simulink library "lib_Transmission"  (R2017b)
settings: Solver=VariableStepAuto  StartTime=0.0  StopTime=10.0  RelTol=1e-3
undefined symbols (not defined in the file): Engine, gb, Gearbox, Loss, Ratio, Spd
libraries: simulink x5
settings Model: Creator=Vraj M  LastModifiedBy=Lyu19
settings CodeAppCC: StateflowObjectComments=on

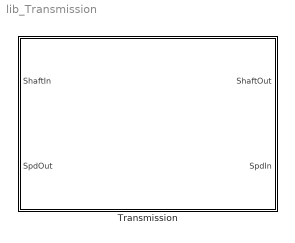
== system lib_Transmission ==
  Transmission : Subsystem
      mask Display:
      | image('Images\Trans.png')
      | color('red');
      | port_label('Input',1,'ShaftIn')
      | port_label('Input',2,'SpdOut')
      | port_label('Output',1,'ShaftOut')
      | port_label('Output',2,'SpdIn')

== system lib_Transmission/Transmission ==
  ShaftIn : Inport
  SpdOut : Inport  Port=2
  Inputs : Subsystem  AncestorBlock=lib_DCDC/DC-DC Converter/Inputs
  Outputs : Subsystem  AncestorBlock=lib_DCDC/DC-DC Converter/Outputs
  Soft TCM : Subsystem
      mask Display: image('softECU.jpg')
  Transmission Plant : Subsystem
      mask Display:
      | image('Images\Trans.png')
      | color('red');
      | port_label('Input',2,'ShaftIn')
      | port_label('Input',3,'SpdOut')
      | port_label('Output',2,'ShaftOut')
      | port_label('Output',3,'SpdIn')
  ShaftOut : Outport
  SpdIn : Outport  Port=2
  wires:
  Transmission Plant/3(TorqConvSpdIn) -> SpdIn/1
  Transmission Plant/2(GearboxShaftOut) -> ShaftOut/1
  SpdOut/1 -> Transmission Plant/3(GearboxSpdOut)
  ShaftIn/1 -> Transmission Plant/2(TorqConvShaftIn)
  Soft TCM/1(Out) -> Outputs/1(Outputs)
  Inputs/1(Inputs) -> Soft TCM/1(In)
  Transmission Plant/1(Out1) -> Soft TCM/2(In1)  "Sensors_to_TCM"
  Soft TCM/2(Out1) -> Transmission Plant/1("In1 ")  "TCM_to_Actuators"

== system lib_Transmission/Transmission/Inputs ==
  Analog_fromHCU : Subsystem
  Bus Creator1 : BusCreator  Inputs=3
  CAN_fromHCU : Subsystem
  Digital_fromHCU : Subsystem
  Inputs : Outport
  wires:
  Digital_fromHCU/1(Outputs) -> Bus Creator1/2  "Digital"
  CAN_fromHCU/1(Outputs) -> Bus Creator1/1  "CAN"
  Bus Creator1/1 -> Inputs/1
  Analog_fromHCU/1(Outputs) -> Bus Creator1/3

== system lib_Transmission/Transmission/Outputs ==
  Outputs : Inport
  tag scope: TCM_to_HCU=global
  wires:
  Outputs/1 -> [TCM_to_HCU]  "TCM_CAN"

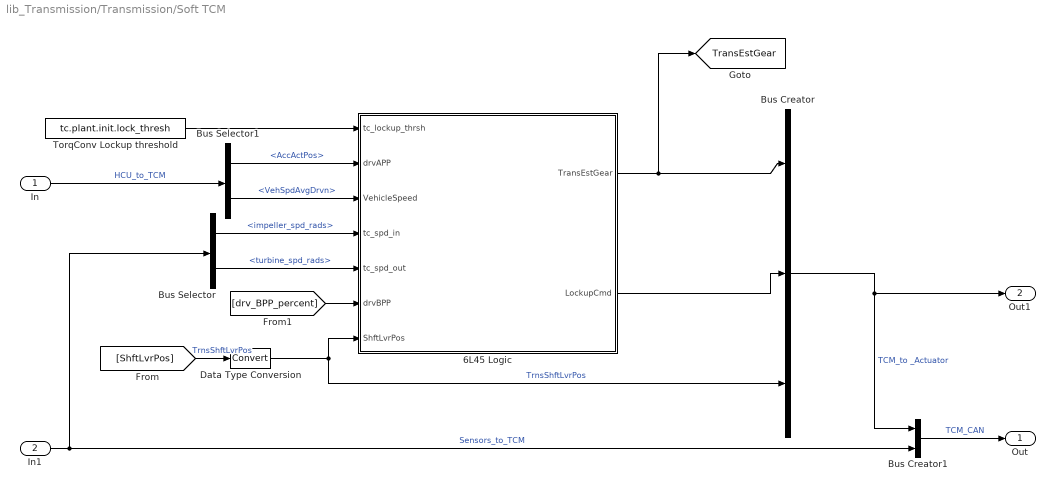
== system lib_Transmission/Transmission/Soft TCM ==
  In : Inport
  In1 : Inport  Port=2
  6L45 Logic : Stateflow chart  TreatAsAtomicUnit=on
  Bus Creator : BusCreator  Inputs=3
  Bus Creator1 : BusCreator  Inputs=2
  Bus Selector : BusSelector  OutputSignals=impeller_spd_rads,turbine_spd_rads
  Bus Selector1 : BusSelector  OutputSignals=CAN.PPEI_Engine_General_Status_1.AccActPos,CAN.PPEI_Vehicle_Speed_and_Distance.VehSpdAvgDrvn
  Data Type Conversion : DataTypeConversion
  TorqConv Lockup threshold : Constant  Value=tc.plant.init.lock_thresh
  Out : Outport
  Out1 : Outport  Port=2
  tag scope: TransEstGear=global
  wires:
  TorqConv Lockup threshold/1 -> 6L45 Logic/1(tc_lockup_thrsh)
  6L45 Logic/1(TransEstGear) -> [TransEstGear], Bus Creator/1
  Data Type Conversion/1 -> Bus Creator/3, 6L45 Logic/7(ShftLvrPos)  "TrnsShftLvrPos"
  In1/1 -> Bus Selector/1, Bus Creator1/2  "Sensors_to_TCM"
  Bus Creator1/1 -> Out/1  "TCM_CAN"
  In/1 -> Bus Selector1/1  "HCU_to_TCM"
  Bus Selector/2 -> 6L45 Logic/5(tc_spd_out)  "<turbine_spd_rads>"
  Bus Selector/1 -> 6L45 Logic/4(tc_spd_in)  "<impeller_spd_rads>"
  Bus Selector1/2 -> 6L45 Logic/3(VehicleSpeed)  "<VehSpdAvgDrvn>"
  Bus Selector1/1 -> 6L45 Logic/2(drvAPP)  "<AccActPos>"
  Bus Creator/1 -> Out1/1, Bus Creator1/1  "TCM_to _Actuator"
  6L45 Logic/2(LockupCmd) -> Bus Creator/2
  [drv_BPP_percent] -> 6L45 Logic/6(drvBPP)
  [ShftLvrPos] -> Data Type Conversion/1  "TrnsShftLvrPos"

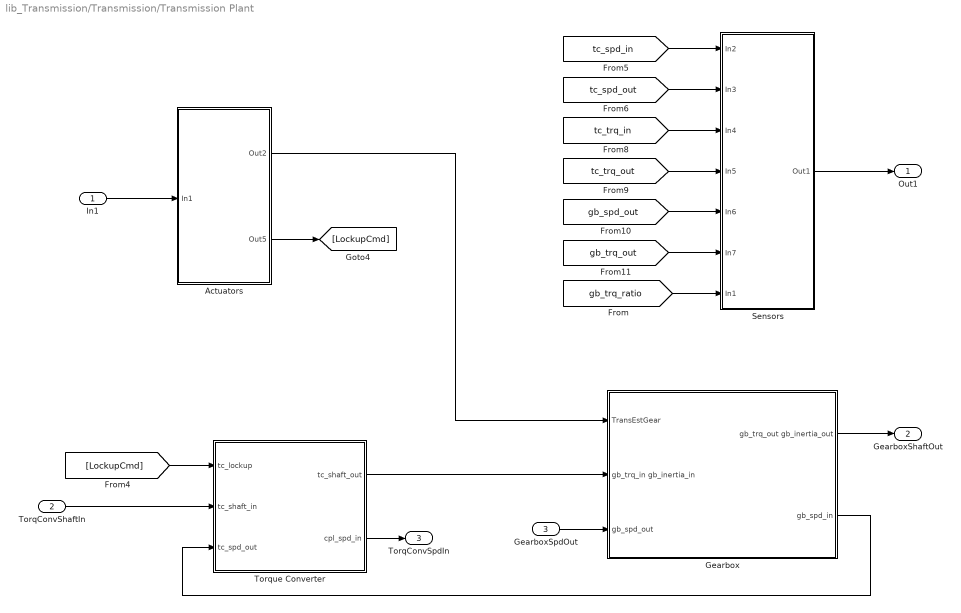
== system lib_Transmission/Transmission/Transmission Plant ==
  "In1 " : Inport
  TorqConvShaftIn : Inport  Port=2
  GearboxSpdOut : Inport  Port=3
  " Actuators" : Subsystem
  Gearbox : Subsystem
      mask Display:
      | image('Images\Gearbox.jpg')
      | color('red');
      | port_label('Input',1,'Gear');
      | port_label('Input',2,'ShftIn');
      | port_label('Input',3,'SpdOut');
      | port_label('Output',1,'ShaftOut');
      | port_label('Output',2,'SpdIn');
  Sensors : Subsystem
  Torque Converter : Subsystem
      mask Display:
      | image('Images\TorqConv.jpg')
      | color('red');
      | port_label('Input',2,'ShaftIn');
      | port_label('Input',3,'SpdOut');
      | port_label('Output',1,'ShaftOut');
      | port_label('Output',2,'SpdIn');
  Out1 : Outport
  GearboxShaftOut : Outport  Port=2
  TorqConvSpdIn : Outport  Port=3
  wires:
  [tc_trq_out] -> Sensors/4(In5)
  [gb_spd_out] -> Sensors/5(In6)
  [gb_trq_out] -> Sensors/6(In7)
  [tc_spd_out] -> Sensors/2(In3)
  [tc_spd_in] -> Sensors/1(In2)
  [tc_trq_in] -> Sensors/3(In4)
  " Actuators"/2(Out5) -> [LockupCmd]
  "In1 "/1 -> " Actuators"/1(In1)
  Sensors/1(Out1) -> Out1/1
  [gb_trq_ratio] -> Sensors/7(In1)
  Torque Converter/2(cpl_spd_in) -> TorqConvSpdIn/1
  Gearbox/2(gb_spd_in) -> Torque Converter/3(tc_spd_out)
  TorqConvShaftIn/1 -> Torque Converter/2(tc_shaft_in)
  Gearbox/1(gb_trq_out gb_inertia_out) -> GearboxShaftOut/1
  " Actuators"/1(Out2) -> Gearbox/1(TransEstGear)
  Torque Converter/1(tc_shaft_out) -> Gearbox/2(gb_trq_in gb_inertia_in)
  GearboxSpdOut/1 -> Gearbox/3(gb_spd_out)
  [LockupCmd] -> Torque Converter/1(tc_lockup)

== system lib_Transmission/Transmission/Inputs/Analog_fromHCU ==
  Outputs : Outport
  wires:
  [Analog] -> Outputs/1

== system lib_Transmission/Transmission/Inputs/CAN_fromHCU ==
  Outputs : Outport
  wires:
  [HCU_to_VEH_CAN] -> Outputs/1

== system lib_Transmission/Transmission/Inputs/Digital_fromHCU ==
  Outputs : Outport
  wires:
  [Digital] -> Outputs/1

== system lib_Transmission/Transmission/Soft TCM/6L45 Logic/Gearbox_Control.Shift_Schedule.PlotShiftSchedule ==
  f : TriggerPort  TriggerType=function-call  VariantControl=Variant
      settings: CopyFcn=Stateflow.SLINSF.SimulinkMan.removeBlockPreDeleteFcn  PreDeleteFcn=Stateflow.SLINSF.SimulinkMan.unsafePredeleteFcn
  Subsystem : Subsystem
      settings: OpenFcn=|
      | figure;
      | PlotGearShiftSchedule(Gearbox.L45.PedalPositions,Gearbox.L45.UpShiftSpeeds,Gearbox.L45.DownShiftSpeeds,'6L45')
      mask Display: disp('Plot')

== system lib_Transmission/Transmission/Soft TCM/6L45 Logic/Gearbox_Control.Shift_Schedule.calc_down ==
  Gear : Inport
  APP : Inport  Port=2
  f : TriggerPort  TriggerType=function-call  VariantControl=Variant
      settings: CopyFcn=Stateflow.SLINSF.SimulinkMan.removeBlockPreDeleteFcn  PreDeleteFcn=Stateflow.SLINSF.SimulinkMan.unsafePredeleteFcn
  Calculate Downshift Threshold : Lookup2D  RowIndex=gb.ctrl.dmd.init.gear_dnshift.idx1_lin_accel  ColumnIndex=[2,3,4,5,6,7,8]  Table=gb.ctrl.dmd.init.gear_dnshift.map'  LookUpMeth=Interpolation-Use End Values
  down_th : Outport
  wires:
  APP/1 -> Calculate Downshift Threshold/1
  Gear/1 -> Calculate Downshift Threshold/2
  Calculate Downshift Threshold/1 -> down_th/1

== system lib_Transmission/Transmission/Soft TCM/6L45 Logic/Gearbox_Control.Shift_Schedule.calc_up ==
  Gear : Inport
  APP : Inport  Port=2
  f : TriggerPort  TriggerType=function-call  VariantControl=Variant
      settings: CopyFcn=Stateflow.SLINSF.SimulinkMan.removeBlockPreDeleteFcn  PreDeleteFcn=Stateflow.SLINSF.SimulinkMan.unsafePredeleteFcn
  Calculate Upshift Threshold : Lookup2D  RowIndex=gb.ctrl.dmd.init.gear_upshift.idx1_lin_accel  ColumnIndex=[1,2,3,4,5,6,7]  Table=gb.ctrl.dmd.init.gear_upshift.map'  LookUpMeth=Interpolation-Use End Values
  up_th : Outport
  wires:
  Gear/1 -> Calculate Upshift Threshold/2
  APP/1 -> Calculate Upshift Threshold/1
  Calculate Upshift Threshold/1 -> up_th/1

== system lib_Transmission/Transmission/Soft TCM/6L45 Logic/Torque_Converter_Control.calc_lockup ==
  Gear : Inport
  APP : Inport  Port=2
  f : TriggerPort  TriggerType=function-call  VariantControl=Variant
      settings: CopyFcn=Stateflow.SLINSF.SimulinkMan.removeBlockPreDeleteFcn  PreDeleteFcn=Stateflow.SLINSF.SimulinkMan.unsafePredeleteFcn
  Calculate Lockup Threshold : Lookup2D  RowIndex=cpl.ctrl.init.trqconv_lockup.idx1_lin_accel  ColumnIndex=cpl.ctrl.init.trqconv_lockup.idx2_gear  Table=cpl.ctrl.init.trqconv_lockup.map  LookUpMeth=Interpolation-Use End Values
  lockup_th : Outport
  wires:
  Gear/1 -> Calculate Lockup Threshold/2
  APP/1 -> Calculate Lockup Threshold/1
  Calculate Lockup Threshold/1 -> lockup_th/1

== system lib_Transmission/Transmission/Soft TCM/6L45 Logic/Torque_Converter_Control.calc_unlock ==
  Gear : Inport
  APP : Inport  Port=2
  f : TriggerPort  TriggerType=function-call  VariantControl=Variant
      settings: CopyFcn=Stateflow.SLINSF.SimulinkMan.removeBlockPreDeleteFcn  PreDeleteFcn=Stateflow.SLINSF.SimulinkMan.unsafePredeleteFcn
  Calculate Unlock Threshold : Lookup2D  RowIndex=cpl.ctrl.init.trqconv_unlock.idx1_lin_accel  ColumnIndex=cpl.ctrl.init.trqconv_unlock.idx2_gear  Table=cpl.ctrl.init.trqconv_unlock.map  LookUpMeth=Interpolation-Use End Values
  unlock_th : Outport
  wires:
  Gear/1 -> Calculate Unlock Threshold/2
  APP/1 -> Calculate Unlock Threshold/1
  Calculate Unlock Threshold/1 -> unlock_th/1

== system lib_Transmission/Transmission/Transmission Plant/ Actuators ==
  In1 : Inport
  Bus Selector : BusSelector  OutputSignals=TransEstGear,LockupCmd
  Out2 : Outport
  Out5 : Outport  Port=2
  wires:
  Bus Selector/2 -> Out5/1  "<LockupCmd>"
  Bus Selector/1 -> Out2/1  "<TransEstGear>"
  In1/1 -> Bus Selector/1

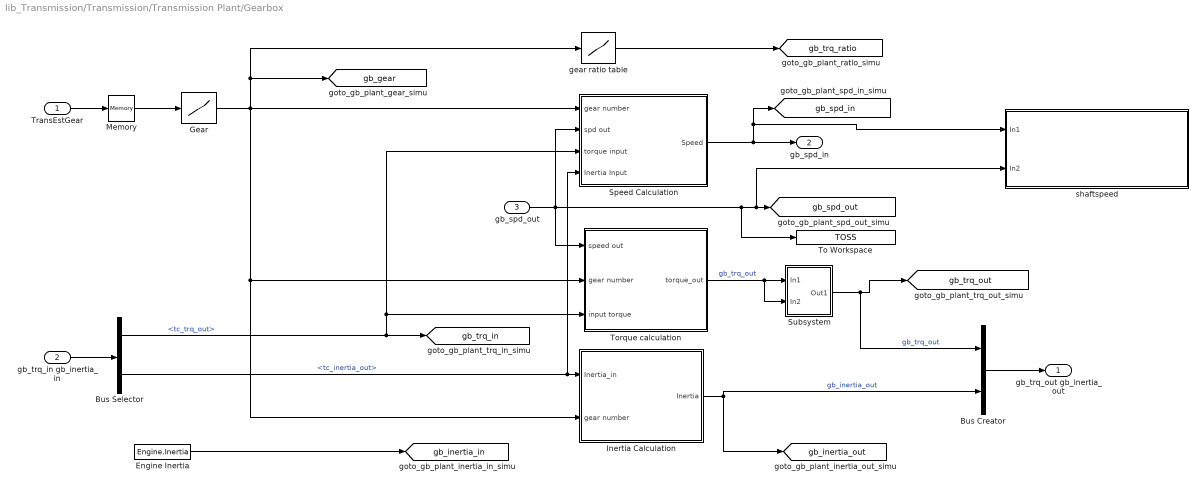
== system lib_Transmission/Transmission/Transmission Plant/Gearbox ==
  TransEstGear : Inport
  gb_trq_in gb_inertia_in : Inport  Port=2
  gb_spd_out : Inport  Port=3
  Bus Creator : BusCreator  Inputs=2
  Bus Selector : BusSelector  OutputSignals=tc_trq_out,tc_inertia_out
  Engine Inertia : Constant  Value=Engine.Inertia
  Gear : Lookup  InputValues=gb.plant.init.gear.idx1_shifter  Table=gb.plant.init.gear.idx2_gear  LookUpMeth=Interpolation-Use End Values  OutDataTypeStr=double  SaturateOnIntegerOverflow=on
  Inertia Calculation : Subsystem
  Memory : Memory
  Speed Calculation : Subsystem
  Subsystem : Subsystem
  To Workspace : ToWorkspace  VariableName=TOSS  SampleTime=-1
  Torque calculation : Subsystem
  gear ratio table : Lookup  InputValues=gb.plant.init.ratio.idx1_gear  Table=gb.plant.init.ratio.map  LookUpMeth=Interpolation-Use End Values  SaturateOnIntegerOverflow=on
  "shaftspeed " : Subsystem
  gb_trq_out gb_inertia_out : Outport
  gb_spd_in : Outport  Port=2
  tag scope: gb_gear=global, gb_inertia_in=global, gb_inertia_out=global, gb_spd_in=global, gb_spd_out=global, gb_trq_in=global, gb_trq_out=global, gb_trq_ratio=global
  wires:
  TransEstGear/1 -> Memory/1
  Bus Selector/1 -> [gb_trq_in], Speed Calculation/3(torque input), Torque calculation/3(" input torque")  "<tc_trq_out>"
  Gear/1 -> Speed Calculation/1(gear number), [gb_gear], gear ratio table/1, Inertia Calculation/2(gear number), Torque calculation/2(gear number)
  gb_spd_out/1 -> Torque calculation/1(speed out), To Workspace/1, "shaftspeed "/2(In2), [gb_spd_out], Speed Calculation/2(spd out)
  gb_trq_in gb_inertia_in/1 -> Bus Selector/1
  Speed Calculation/1(Speed) -> "shaftspeed "/1(In1), [gb_spd_in], gb_spd_in/1
  Inertia Calculation/1(Inertia) -> [gb_inertia_out], Bus Creator/2  "gb_inertia_out"
  Bus Creator/1 -> gb_trq_out gb_inertia_out/1
  gear ratio table/1 -> [gb_trq_ratio]
  Memory/1 -> Gear/1
  Torque calculation/1(torque_out) -> Subsystem/2(In2), Subsystem/1(In1)  "gb_trq_out"
  Subsystem/1(Out1) -> Bus Creator/1, [gb_trq_out]  "gb_trq_out"
  Engine Inertia/1 -> [gb_inertia_in]
  Bus Selector/2 -> Speed Calculation/4(Inertia Input), Inertia Calculation/1(Inertia_in)  "<tc_inertia_out>"

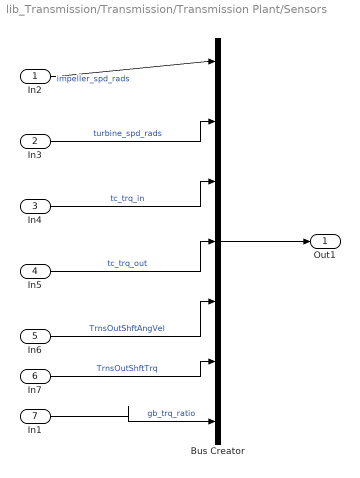
== system lib_Transmission/Transmission/Transmission Plant/Sensors ==
  In2 : Inport
  In3 : Inport  Port=2
  In4 : Inport  Port=3
  In5 : Inport  Port=4
  In6 : Inport  Port=5
  In7 : Inport  Port=6
  In1 : Inport  Port=7
  Bus Creator : BusCreator  Inputs=7
  Out1 : Outport
  wires:
  In7/1 -> Bus Creator/6  "TrnsOutShftTrq"
  In6/1 -> Bus Creator/5  "TrnsOutShftAngVel"
  In3/1 -> Bus Creator/2  "turbine_spd_rads"
  In5/1 -> Bus Creator/4  "tc_trq_out"
  In4/1 -> Bus Creator/3  "tc_trq_in"
  In2/1 -> Bus Creator/1  "impeller_spd_rads"
  Bus Creator/1 -> Out1/1
  In1/1 -> Bus Creator/7  "gb_trq_ratio"

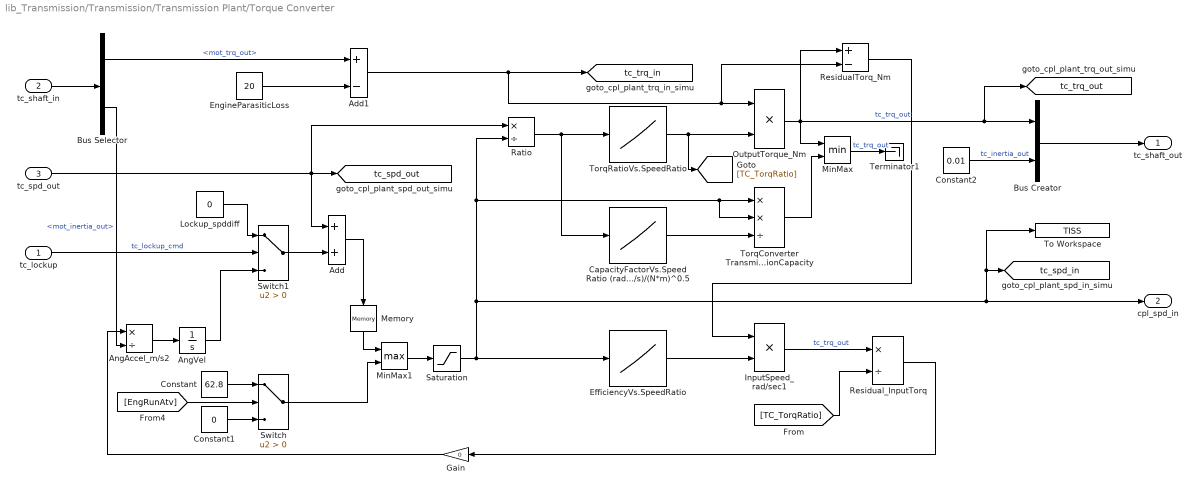
== system lib_Transmission/Transmission/Transmission Plant/Torque Converter ==
  tc_lockup : Inport
  tc_shaft_in : Inport  Port=2
  tc_spd_out : Inport  Port=3
  Add : Sum
  Add1 : Sum  Inputs=+-
  AngAccel_m/s2 : Product  Inputs=*/
  AngVel : Integrator
  Bus Creator : BusCreator  Inputs=2
  Bus Selector : BusSelector  OutputSignals=mot_trq_out,mot_inertia_out
  CapacityFactorVs.SpeedRatio (rad/s)/(N*m)^0.5 : Lookup_n-D  NumberOfTableDimensions=1  BreakpointsForDimension1=[0 0.50 0.60 0.70 0.80 0.87 0.92 0.94 0.96 0.97]  Table=[12.2938 12.8588 13.1452 13.6285 14.6163 16.2675 19.3503 22.1046 29.9986 50.00]  InternalRulePriority=Speed  RndMeth=Simplest  InputSameDT=on
  Constant : Constant  Value=62.8
  Constant1 : Constant  Value=0
  Constant2 : Constant  Value=0.01
  EfficiencyVs.SpeedRatio : Lookup_n-D  NumberOfTableDimensions=1  BreakpointsForDimension1=[0 0.25 0.50 0.60 0.70 0.80 0.87 0.92 0.94 0.96 0.97 1.0]  Table="[0.10 0.50 0.70 0.8 0.8 0.80  0.85 0.87 0.91 0.95 0.96 0.96]"  InternalRulePriority=Speed  RndMeth=Simplest  InputSameDT=on
  EngineParasiticLoss : Constant  Value=20
  Gain : Gain  Gain=0
  InputSpeed_rad/sec1 : Product  Inputs=**
  Lockup_spddiff : Constant  Value=0
  Memory : Memory  InitialCondition=1
  MinMax : MinMax  Inputs=2
  MinMax1 : MinMax  Function=max  Inputs=2
  OutputTorque_Nm : Product  Inputs=**
  Ratio : Product  Inputs=*/
  ResidualTorq_Nm : Sum  Inputs=+-
  Residual_InputTorq : Product  Inputs=*/
  Saturation : Saturate  UpperLimit=1100  LowerLimit=1
  Switch : Switch  Criteria=u2 > Threshold
  Switch1 : Switch  Criteria=u2 > Threshold
  Terminator1 : Terminator
  To Workspace : ToWorkspace  VariableName=TISS  SampleTime=-1
  TorqConverter TransmissionCapacity : Product  Inputs=**/
  TorqRatioVs.SpeedRatio : Lookup_n-D  NumberOfTableDimensions=1  BreakpointsForDimension1=[0 0.50 0.60 0.70 0.80 0.87 0.92 0.94 0.96 0.97]  Table=[2.2320 1.5462 1.4058 1.2746 1.1528 1.0732 1.0192 0.9983 0.9983 0.9983]  InternalRulePriority=Speed  RndMeth=Simplest  InputSameDT=on
  tc_shaft_out : Outport
  cpl_spd_in : Outport  Port=2
  tag scope: tc_spd_in=global, tc_spd_out=global, tc_trq_in=global, tc_trq_out=global
  wires:
  Add1/1 -> [tc_trq_in], ResidualTorq_Nm/2, OutputTorque_Nm/1
  Constant2/1 -> Bus Creator/2  "tc_inertia_out"
  tc_shaft_in/1 -> Bus Selector/1
  Bus Creator/1 -> tc_shaft_out/1
  Bus Selector/2 -> AngAccel_m/s2/2  "<mot_inertia_out>"
  tc_lockup/1 -> Switch1/2  "tc_lockup_cmd"
  TorqRatioVs.SpeedRatio/1 -> OutputTorque_Nm/2, [TC_TorqRatio]
  CapacityFactorVs.SpeedRatio (rad/s)/(N*m)^0.5/1 -> TorqConverter TransmissionCapacity/3
  Ratio/1 -> CapacityFactorVs.SpeedRatio (rad/s)/(N*m)^0.5/1, TorqRatioVs.SpeedRatio/1
  Saturation/1 -> Ratio/2, TorqConverter TransmissionCapacity/2, TorqConverter TransmissionCapacity/1, [tc_spd_in], To Workspace/1, cpl_spd_in/1, EfficiencyVs.SpeedRatio/1
  EfficiencyVs.SpeedRatio/1 -> InputSpeed_rad/sec1/2
  TorqConverter TransmissionCapacity/1 -> MinMax/2
  [TC_TorqRatio] -> Residual_InputTorq/2
  ResidualTorq_Nm/1 -> InputSpeed_rad/sec1/1
  InputSpeed_rad/sec1/1 -> Residual_InputTorq/1  "tc_trq_out"
  AngAccel_m/s2/1 -> AngVel/1
  AngVel/1 -> Switch1/3
  Memory/1 -> MinMax1/1
  EngineParasiticLoss/1 -> Add1/2
  Residual_InputTorq/1 -> Gain/1
  OutputTorque_Nm/1 -> ResidualTorq_Nm/1, Bus Creator/1, [tc_trq_out], MinMax/1  "tc_trq_out"
  MinMax/1 -> Terminator1/1  "tc_trq_out"
  tc_spd_out/1 -> Ratio/1, [tc_spd_out], Add/1
  Add/1 -> Memory/1
  Gain/1 -> AngAccel_m/s2/1
  MinMax1/1 -> Saturation/1
  Switch/1 -> MinMax1/2
  [EngRunAtv] -> Switch/2
  Constant/1 -> Switch/1
  Constant1/1 -> Switch/3
  Bus Selector/1 -> Add1/1  "<mot_trq_out>"
  Switch1/1 -> Add/2
  Lockup_spddiff/1 -> Switch1/1

== system lib_Transmission/Transmission/Soft TCM/6L45 Logic/Gearbox_Control.Shift_Schedule.PlotShiftSchedule/Subsystem ==

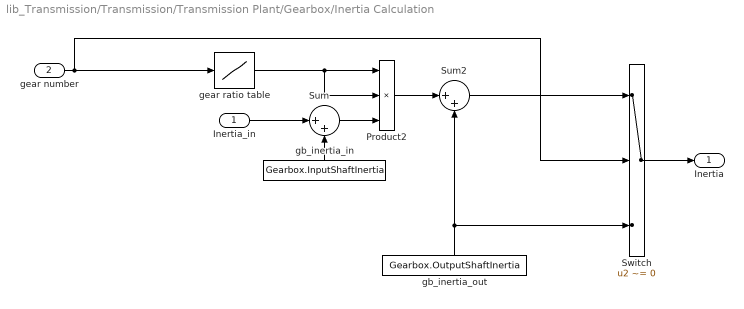
== system lib_Transmission/Transmission/Transmission Plant/Gearbox/Inertia Calculation ==
  Inertia_in : Inport
  gear number : Inport  Port=2
  Product2 : Product  Inputs=3  SaturateOnIntegerOverflow=on  InputSameDT=on  OutDataTypeStr=Inherit: Same as first input
  Sum : Sum  Inputs=|++  SaturateOnIntegerOverflow=on  InputSameDT=on  OutDataTypeStr=Inherit: Same as first input
  Sum2 : Sum  Inputs=|++  SaturateOnIntegerOverflow=on  InputSameDT=on  OutDataTypeStr=Inherit: Same as first input
  Switch : Switch  Criteria=u2 ~= 0  Threshold=0.5  SaturateOnIntegerOverflow=on  InputSameDT=on
  gb_inertia_in : Constant  Value=Gearbox.InputShaftInertia
  gb_inertia_out : Constant  Value=Gearbox.OutputShaftInertia
  gear ratio table : Lookup  InputValues=gb.plant.init.ratio.idx1_gear  Table=gb.plant.init.ratio.map  OutDataTypeStr=double  SaturateOnIntegerOverflow=on
  Inertia : Outport
  wires:
  gear ratio table/1 -> Product2/1, Product2/2
  Sum2/1 -> Switch/1
  Inertia_in/1 -> Sum/1
  Product2/1 -> Sum2/1
  gb_inertia_in/1 -> Sum/2
  Sum/1 -> Product2/3
  gb_inertia_out/1 -> Sum2/2, Switch/3
  gear number/1 -> Switch/2, gear ratio table/1
  Switch/1 -> Inertia/1

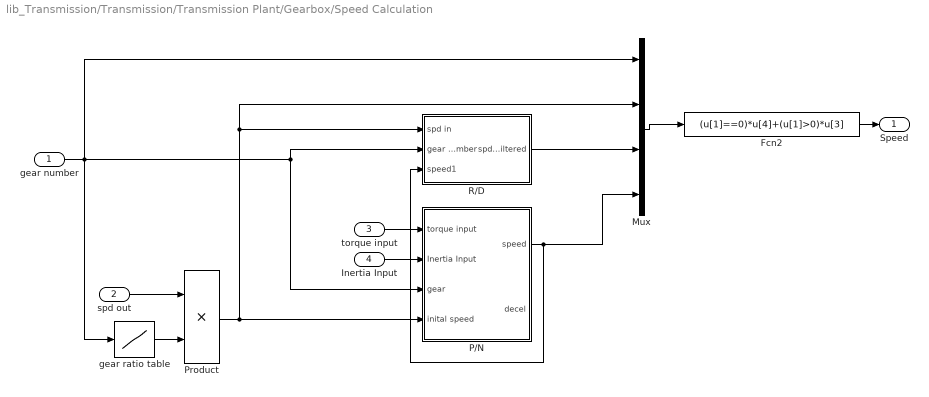
== system lib_Transmission/Transmission/Transmission Plant/Gearbox/Speed Calculation ==
  gear number : Inport
  spd out : Inport  Port=2
  torque input : Inport  Port=3
  Inertia Input : Inport  Port=4
  Fcn2 : Fcn  Expr=(u[1]==0)*u[4]+(u[1]>0)*u[3]
  Mux : Mux
  P/N : Subsystem
  Product : Product  SaturateOnIntegerOverflow=on  InputSameDT=on  OutDataTypeStr=Inherit: Same as first input
  R/D : Subsystem
  gear ratio table : Lookup  InputValues=gb.plant.init.ratio.idx1_gear  Table=gb.plant.init.ratio.map  SaturateOnIntegerOverflow=on
  Speed : Outport
  wires:
  Mux/1 -> Fcn2/1
  gear number/1 -> Mux/1, P/N/3(gear), R/D/2(gear number), gear ratio table/1
  torque input/1 -> P/N/1(torque input)
  Inertia Input/1 -> P/N/2(Inertia Input)
  spd out/1 -> Product/1
  gear ratio table/1 -> Product/2
  Product/1 -> Mux/2, R/D/1(spd in), P/N/4(inital speed)
  P/N/1(speed) -> Mux/4, R/D/3(speed1)
  R/D/1(spd in filtered) -> Mux/3
  Fcn2/1 -> Speed/1

== system lib_Transmission/Transmission/Transmission Plant/Gearbox/Subsystem ==
  In1 : Inport
  In2 : Inport  Port=2
  Add : Sum
  Constant : Constant  Value=200
  Switch2 : Switch  Criteria=u2 > Threshold
  Out1 : Outport
  wires:
  Add/1 -> Switch2/1
  Constant/1 -> Add/1
  [Brk_Flt] -> Switch2/2
  In2/1 -> Switch2/3
  In1/1 -> Add/2
  Switch2/1 -> Out1/1

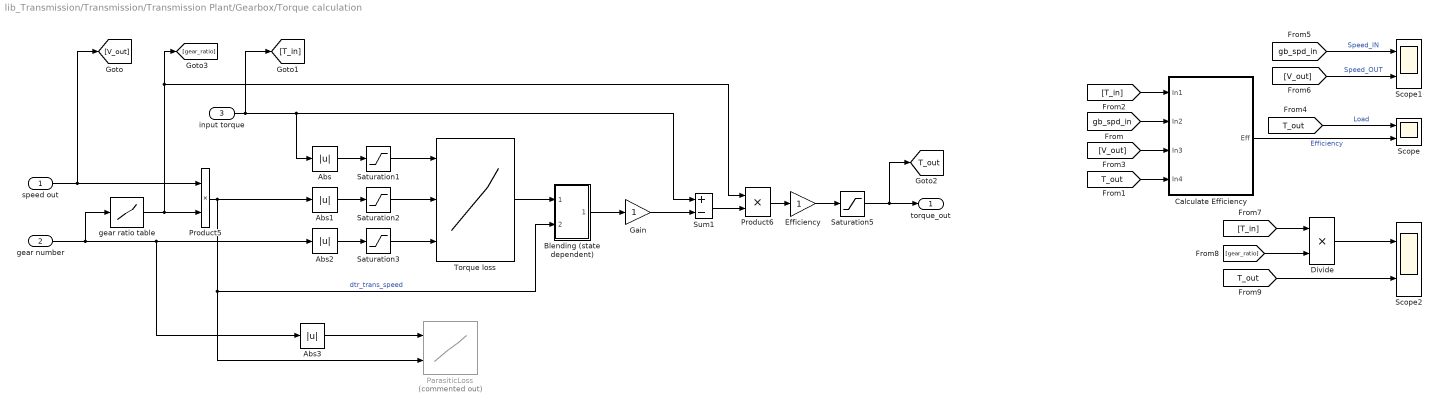
== system lib_Transmission/Transmission/Transmission Plant/Gearbox/Torque calculation ==
  speed out : Inport
  gear number : Inport  Port=2
  " input torque" : Inport  Port=3
  Abs : Abs  SaturateOnIntegerOverflow=on
  Abs1 : Abs  SaturateOnIntegerOverflow=on
  Abs2 : Abs  SaturateOnIntegerOverflow=on
  Abs3 : Abs
  Blending (state dependent) : Subsystem  mask(State dependent blending){xl=-gb.plant.init.spd_thr, yl=-1, xc=0, yc=0, xr=gb.plant.init.spd_thr, yr=1}
      mask prompts: xl "Left point (x):"; yl "Left point (y):"; xc "Center point (x):"; yc "Center point (y):"; xr "Right point (x):"; yr "Right point (y):"
      mask help: This block implements state dependent smoothing/blending. IMPORTANT: See help menu.
      mask Help: The output equals the product of the first input and a "hat" function defined by the three points specified in the dialog box.  The second input forms the argument to the hat function.\n\nIMPORTANT: A divide by zero error will result if first coordinates of the three points specified for the hat function are NOT distinct.
      mask Display: plot([-1 1 3 6 8], [1.5 1.5 0.5 4.0 4.0])
  Calculate Efficiency : Subsystem
  Divide : Product  Inputs=**
  Efficiency : Gain
  Gain : Gain
  ParasiticLoss : Lookup_n-D  Commented=on  BreakpointsForDimension1=Ratio  BreakpointsForDimension2=Spd  Table=Loss  InternalRulePriority=Speed  RndMeth=Simplest  InputSameDT=on
  Product5 : Product  SaturateOnIntegerOverflow=on  InputSameDT=on  OutDataTypeStr=Inherit: Same as first input
  Product6 : Product  SaturateOnIntegerOverflow=on  InputSameDT=on  OutDataTypeStr=Inherit: Same as first input
  Saturation1 : Saturate  UpperLimit=inf  LowerLimit=min( gb.plant.init.trq_loss.idx1_trq )
  Saturation2 : Saturate  UpperLimit=inf  LowerLimit=min( gb.plant.init.trq_loss.idx2_spd )
  Saturation3 : Saturate  UpperLimit=8  LowerLimit=1
  Saturation5 : Saturate  UpperLimit=inf  LowerLimit=min( gb.plant.init.trq_loss.idx1_trq )
  Scope : Scope  NumInputPorts=2
  Scope1 : Scope  NumInputPorts=2
  Scope2 : Scope  NumInputPorts=2
  Sum1 : Sum  Inputs=+-  SaturateOnIntegerOverflow=on  InputSameDT=on  OutDataTypeStr=Inherit: Same as first input
  Torque loss : Lookup_n-D  NumberOfTableDimensions=3  BreakpointsForDimension1=gb.plant.init.trq_loss.idx1_trq  BreakpointsForDimension2=gb.plant.init.trq_loss.idx2_spd  BreakpointsForDimension3=gb.plant.init.trq_loss.idx3_gear  Table=gb.plant.init.trq_loss.map
  gear ratio table : Lookup  InputValues=gb.plant.init.ratio.idx1_gear  Table=gb.plant.init.ratio.map  SaturateOnIntegerOverflow=on
  torque_out : Outport
  tag scope: T_out=global
  wires:
  Saturation2/1 -> Torque loss/2
  Saturation1/1 -> Torque loss/1
  Abs/1 -> Saturation1/1
  Product5/1 -> ParasiticLoss/2, Blending (state dependent)/2(Control (state)), Abs1/1  "dtr_trans_speed"
  Abs1/1 -> Saturation2/1
  speed out/1 -> [V_out], Product5/1
  Product6/1 -> Efficiency/1
  Blending (state dependent)/1(Output) -> Gain/1
  Sum1/1 -> Product6/2
  " input torque"/1 -> [T_in], Sum1/1, Abs/1
  gear number/1 -> Abs3/1, Abs2/1, gear ratio table/1
  gear ratio table/1 -> Product5/2, [gear_ratio], Product6/1
  Abs2/1 -> Saturation3/1
  Saturation3/1 -> Torque loss/3
  Abs3/1 -> ParasiticLoss/1
  Efficiency/1 -> Saturation5/1
  Gain/1 -> Sum1/2
  Torque loss/1 -> Blending (state dependent)/1(Input)
  [T_in] -> Calculate Efficiency/1(In1)
  [gb_spd_in] -> Calculate Efficiency/2(In2)
  [T_out] -> Calculate Efficiency/4(In4)
  Calculate Efficiency/1(Eff) -> Scope/2  "Efficiency"
  [V_out] -> Calculate Efficiency/3(In3)
  [T_out] -> Scope/1  "Load"
  [gb_spd_in] -> Scope1/1  "Speed_IN"
  [V_out] -> Scope1/2  "Speed_OUT"
  [T_in] -> Divide/1
  [gear_ratio] -> Divide/2
  Divide/1 -> Scope2/1
  [T_out] -> Scope2/2
  Saturation5/1 -> torque_out/1, [T_out]

== system lib_Transmission/Transmission/Transmission Plant/Gearbox/shaftspeed  ==
  In1 : Inport
  In2 : Inport  Port=2
  Gain : Gain  Gain=30/pi
  Gain1 : Gain  Gain=30/pi
  Rate Transition1 : RateTransition  OutPortSampleTime=1
  Rate Transition7 : RateTransition  OutPortSampleTime=1
  To Workspace3 : ToWorkspace  VariableName=TrnsOutShftAngVel  SampleTime=-1
  To Workspace4 : ToWorkspace  VariableName=TrnTrbAngVl  SampleTime=-1
  wires:
  In2/1 -> Gain1/1
  In1/1 -> Gain/1
  Gain/1 -> Rate Transition7/1
  Rate Transition7/1 -> To Workspace4/1
  Rate Transition1/1 -> To Workspace3/1
  Gain1/1 -> Rate Transition1/1

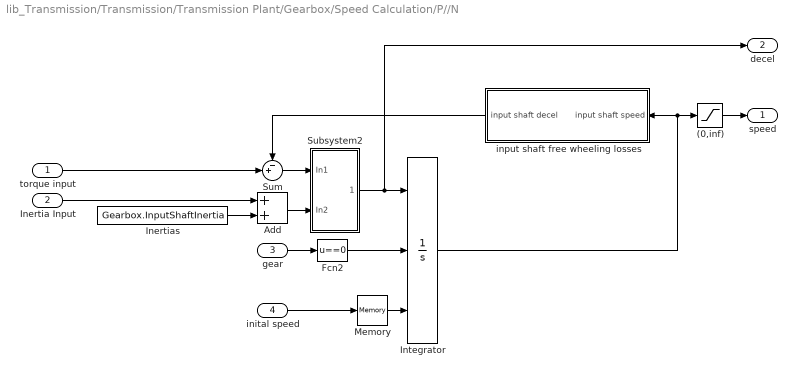
== system lib_Transmission/Transmission/Transmission Plant/Gearbox/Speed Calculation/P//N ==
  torque input : Inport
  Inertia Input : Inport  Port=2
  gear : Inport  Port=3
  inital speed : Inport  Port=4
  (0,inf) : Saturate  UpperLimit=1100  LowerLimit=0
  Add : Sum
  Fcn2 : Fcn  Expr=u==0
  Inertias : Constant  Value=Gearbox.InputShaftInertia
  Integrator : Integrator  ExternalReset=rising  InitialConditionSource=external
  Memory : Memory
  Subsystem2 : Subsystem
      mask Display: disp('divider')
  Sum : Sum  Inputs=-+|  SaturateOnIntegerOverflow=on  InputSameDT=on  OutDataTypeStr=Inherit: Same as first input
  input shaft free wheeling losses : Subsystem
  speed : Outport
  decel : Outport  Port=2
  wires:
  Inertia Input/1 -> Add/1
  Subsystem2/1(Out1) -> decel/1, Integrator/1
  Memory/1 -> Integrator/3
  (0,inf)/1 -> speed/1
  torque input/1 -> Sum/2
  Sum/1 -> Subsystem2/1(In1)
  input shaft free wheeling losses/1(input shaft decel) -> Sum/1
  Integrator/1 -> input shaft free wheeling losses/1(input shaft speed), (0,inf)/1
  gear/1 -> Fcn2/1
  inital speed/1 -> Memory/1
  Fcn2/1 -> Integrator/2
  Add/1 -> Subsystem2/2(In2)
  Inertias/1 -> Add/2

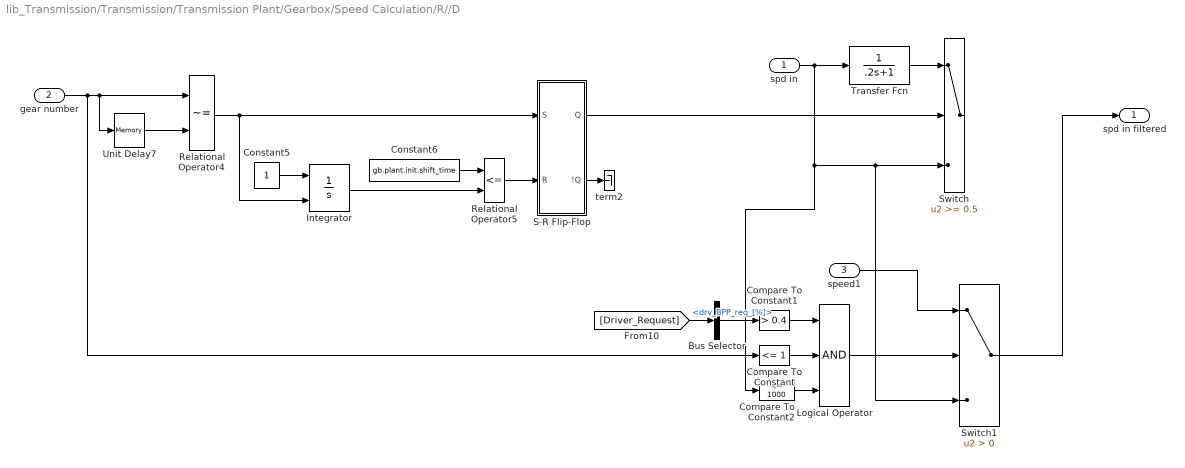
== system lib_Transmission/Transmission/Transmission Plant/Gearbox/Speed Calculation/R//D ==
  spd in : Inport
  gear number : Inport  Port=2
  speed1 : Inport  Port=3
  Bus Selector : BusSelector  OutputSignals=drv_BPP_req_[%]
  Compare To Constant : simulink/Logic and Bit Operations/Compare To Constant  relop=<=  const=1  OutDataTypeStr=boolean
  Compare To Constant1 : simulink/Logic and Bit Operations/Compare To Constant  relop=>  const=0.4  OutDataTypeStr=boolean
  Compare To Constant2 : simulink/Logic and Bit Operations/Compare To Constant  relop=<=  const=1000  OutDataTypeStr=boolean
  Constant5 : Constant
  Constant6 : Constant  Value=gb.plant.init.shift_time
  Integrator : Integrator  ExternalReset=rising
  Logical Operator : Logic  Inputs=3  AllPortsSameDT=off  OutDataTypeStr=boolean
  Relational Operator4 : RelationalOperator  Operator=~=  RndMeth=Nearest  InputSameDT=on
  Relational Operator5 : RelationalOperator  Operator=<=  RndMeth=Nearest  InputSameDT=on
  S-R Flip-Flop : Subsystem  mask(SRFlipFlop){initial_condition=0}
      mask prompts: initial_condition "Initial condition:"
      mask help: S-R Flip Flop Block
  Switch : Switch  Threshold=0.5  SaturateOnIntegerOverflow=on  InputSameDT=on
  Switch1 : Switch  Criteria=u2 > Threshold
  Transfer Fcn : TransferFcn  Denominator=[.2 1]
  Unit Delay7 : Memory
  term2 : Terminator
  spd in filtered : Outport
  wires:
  spd in/1 -> Transfer Fcn/1, Switch/3, Switch1/3, Compare To Constant2/1
  Relational Operator5/1 -> S-R Flip-Flop/2(R)
  S-R Flip-Flop/1(Q) -> Switch/2
  Integrator/1 -> Relational Operator5/2
  Relational Operator4/1 -> S-R Flip-Flop/1(S), Integrator/2
  Unit Delay7/1 -> Relational Operator4/2
  S-R Flip-Flop/2(!Q) -> term2/1
  Constant6/1 -> Relational Operator5/1
  Constant5/1 -> Integrator/1
  gear number/1 -> Compare To Constant/1, Unit Delay7/1, Relational Operator4/1
  [Driver_Request] -> Bus Selector/1
  Bus Selector/1 -> Compare To Constant1/1  "<drv_BPP_req_[%]>"
  Compare To Constant1/1 -> Logical Operator/1
  Compare To Constant/1 -> Logical Operator/2
  Logical Operator/1 -> Switch1/2
  Compare To Constant2/1 -> Logical Operator/3
  Switch1/1 -> spd in filtered/1
  speed1/1 -> Switch1/1
  Transfer Fcn/1 -> Switch/1

== system lib_Transmission/Transmission/Transmission Plant/Gearbox/Torque calculation/Blending (state dependent) ==
  Input : Inport
  Control (state) : Inport  Port=2
  Linear spline : Fcn  Expr=(u<xl)*yl + (xl<=u)*(u<xc)*((yc-yl)*(u-xl)/(xc-xl)+yl) + (xc<=u)*(u<xr)*((yc-yr)*(u-xr)/(xc-xr)+yr) + (xr<=u)*yr
  Product2 : Product  SaturateOnIntegerOverflow=on  InputSameDT=on  OutDataTypeStr=Inherit: Same as first input
  Output : Outport
  wires:
  Control (state)/1 -> Linear spline/1
  Product2/1 -> Output/1
  Linear spline/1 -> Product2/2
  Input/1 -> Product2/1

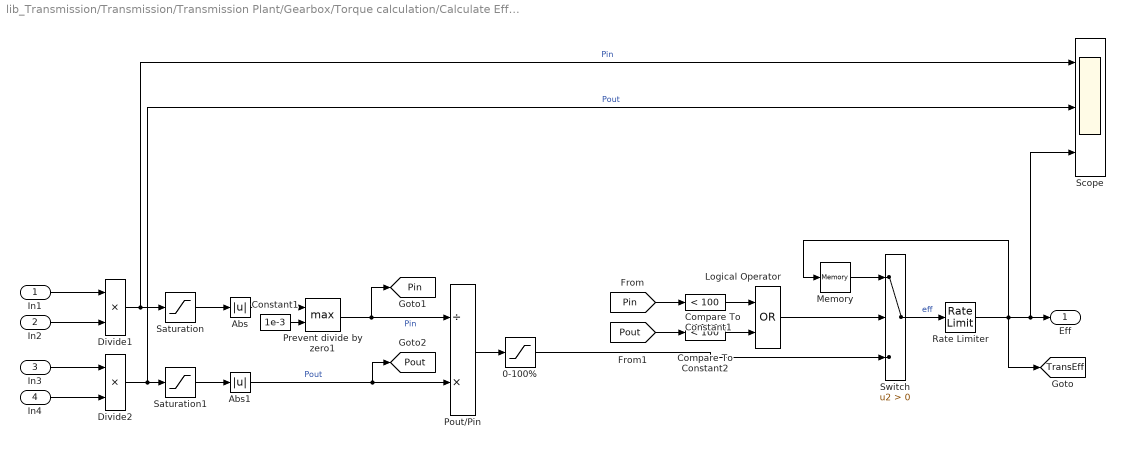
== system lib_Transmission/Transmission/Transmission Plant/Gearbox/Torque calculation/Calculate Efficiency ==
  In1 : Inport
  In2 : Inport  Port=2
  In3 : Inport  Port=3
  In4 : Inport  Port=4
  0-100% : Saturate  UpperLimit=1  LowerLimit=-1
  Abs : Abs
  Abs1 : Abs
  Compare To Constant1 : simulink/Logic and Bit Operations/Compare To Constant  relop=<  const=100  OutDataTypeStr=boolean
  Compare To Constant2 : simulink/Logic and Bit Operations/Compare To Constant  relop=<  const=100  OutDataTypeStr=boolean
  Constant1 : Constant  Value=1e-3
  Divide1 : Product  Inputs=**
  Divide2 : Product  Inputs=**
  Logical Operator : Logic  Operator=OR  AllPortsSameDT=off  OutDataTypeStr=boolean
  Memory : Memory
  Pout/Pin : Product  Inputs=/*
  Prevent divide by zero1 : MinMax  Function=max  Inputs=2
  Rate Limiter : RateLimiter  FallingSlewLimit=-1e-1  SampleTimeMode=inherited
  Saturation : Saturate  UpperLimit=inf  LowerLimit=0
  Saturation1 : Saturate  UpperLimit=inf  LowerLimit=0
  Scope : Scope  NumInputPorts=3
  Switch : Switch  Criteria=u2 > Threshold
  Eff : Outport
  tag scope: Pin=global, Pout=global, TransEff=global
  wires:
  Pout/Pin/1 -> 0-100%/1
  Divide1/1 -> Scope/1, Saturation/1  "Pin"
  Divide2/1 -> Scope/2, Saturation1/1  "Pout"
  In2/1 -> Divide1/2
  In4/1 -> Divide2/2
  In1/1 -> Divide1/1
  In3/1 -> Divide2/1
  Abs/1 -> Prevent divide by zero1/1
  Constant1/1 -> Prevent divide by zero1/2
  Abs1/1 -> Pout/Pin/2, [Pout]  "Pout"
  Prevent divide by zero1/1 -> Pout/Pin/1, [Pin]  "Pin"
  [Pout] -> Compare To Constant2/1
  Logical Operator/1 -> Switch/2
  Switch/1 -> Rate Limiter/1  "eff"
  Memory/1 -> Switch/1
  Saturation/1 -> Abs/1
  Saturation1/1 -> Abs1/1
  [Pin] -> Compare To Constant1/1
  Compare To Constant1/1 -> Logical Operator/1
  Compare To Constant2/1 -> Logical Operator/2
  Rate Limiter/1 -> Memory/1, Scope/3, Eff/1, [TransEff]
  0-100%/1 -> Switch/3

== system lib_Transmission/Transmission/Transmission Plant/Gearbox/Speed Calculation/P//N/Subsystem2 ==
  In1 : Inport
  In2 : Inport  Port=2
  Fcn : Fcn  Expr=u[1]/(u[2]+eps)*(u[2]!=0)
  Mux : Mux  Inputs=2
  Out1 : Outport
  wires:
  Mux/1 -> Fcn/1
  In1/1 -> Mux/1
  Fcn/1 -> Out1/1
  In2/1 -> Mux/2

== system lib_Transmission/Transmission/Transmission Plant/Gearbox/Speed Calculation/P//N/input shaft free wheeling losses ==
  input shaft speed : Inport
  Constant1 : Constant  Value=0
  Fcn1 : Fcn  Expr=u==0
  Gain1 : Gain  Gain=0.15  SaturateOnIntegerOverflow=on  OutDataTypeStr=Inherit: Same as input  ParamDataTypeStr=Inherit: Same as input
  Switch2 : Switch  Threshold=0.5  SaturateOnIntegerOverflow=on  InputSameDT=on
  input shaft decel : Outport
  wires:
  input shaft speed/1 -> Switch2/3, Fcn1/1
  Fcn1/1 -> Switch2/2
  Gain1/1 -> input shaft decel/1
  Switch2/1 -> Gain1/1
  Constant1/1 -> Switch2/1

== system lib_Transmission/Transmission/Transmission Plant/Gearbox/Speed Calculation/R//D/S-R Flip-Flop ==
  S : Inport
  R : Inport  Port=2
  Demux : Demux  Outputs=2
  Logic : CombinatorialLogic  TruthTable=[0 1;0 1;1 0;0 1;1 0;0 1;1 0;1 0]
  Memory : Memory  InitialCondition=initial_condition  InheritSampleTime=on
  Mux : Mux  Inputs=3
  Q : Outport  InitialOutput=0
  !Q : Outport  Port=2  InitialOutput=1
  wires:
  R/1 -> Mux/3
  S/1 -> Mux/2
  Memory/1 -> Mux/1
  Demux/1 -> Memory/1, Q/1
  Demux/2 -> !Q/1
  Logic/1 -> Demux/1
  Mux/1 -> Logic/1

== stateflow chart lib_Transmission/Transmission/Soft TCM/6L45 Logic ==
  settings: sampleTime=0.04
  state Torque_Converter_Control [parallel]
    du:
    du:[lockup_thrsh]=calc_lockup(Gear_D, drvAPP);
    du:[unlock_thrsh]=calc_unlock(Gear_D, drvAPP);
    settings: executionOrder=1
    state lockup_th = calc_lockup(Gear, APP) [function]
    note: Lever Position:
        | 1 P
        | 2 R
        | 3 N
        | 4 D
        |
        | 1 clutch lock-up
        | 0 clutch unlock
    state Lock
      en:
      LockupCmd = 1;
    state Unlock
      en:
      LockupCmd = 0;
    state unlock_th = calc_unlock(Gear,APP) [function]
    (default) -> Unlock
    Unlock -> Lock : [(Gear_D >= 4 || drvBPP > 0) && VehicleSpeed > 20]
    Lock -> Unlock : [VehicleSpeed < 20 || drvBPP == 0 && drvAPP > 5 && Gear_D <= 3]
  state Gearbox_Control [parallel]
    settings: executionOrder=2
    state Shifter_Actuator [parallel]
      settings: executionOrder=1
      state Shifter_D
        du:
        TransEstGear = Gear_D;
      state Shifter_R
        en:
        TransEstGear = 14;
      state Shifter_N
        en:
        TransEstGear = 13;
      state Shifter_P
        en:
        TransEstGear = 15;
      (default) -> Shifter_P
      Shifter_D -> Shifter_N : [ShftLvrPos <= 3]
      Shifter_N -> Shifter_R [order 2] : [ShftLvrPos <= 2]
      Shifter_R -> Shifter_P [order 2] : [ShftLvrPos <= 1]
      Shifter_N -> Shifter_D [order 1] : [ShftLvrPos >= 4]
      Shifter_R -> Shifter_N [order 1] : [ShftLvrPos >= 3]
      Shifter_P -> Shifter_R : [ShftLvrPos >= 2]
    state Shift_Schedule [parallel]
      settings: executionOrder=2
      state Gear_State_D [parallel]
        settings: executionOrder=1
        state Gear_4th
          entry:
          Gear_D = 4;
        state Gear_3rd
          entry:
          Gear_D = 3;
        state Gear_6th
          entry:
          Gear_D = 6;
        state Gear_7th
          entry:
          Gear_D = 7;
        state Gear_8th
          entry:
          Gear_D = 8;
        state Gear_1st
          entry:
          Gear_D = 1;
        state Gear_5th
          entry:
          Gear_D = 5;
        state Gear_2nd
          entry:
          Gear_D  = 2;
        (default) -> Gear_1st
        Gear_2nd -> Gear_3rd [order 1] : UP
        Gear_7th -> Gear_8th [order 1] : UP
        Gear_4th -> Gear_5th [order 1] : UP
        Gear_5th -> Gear_6th [order 1] : UP
        Gear_6th -> Gear_7th [order 1] : UP
        Gear_3rd -> Gear_4th [order 1] : UP
        Gear_1st -> Gear_2nd : UP
        Gear_3rd -> Gear_2nd [order 2] : DOWN
        Gear_4th -> Gear_3rd [order 2] : DOWN
        Gear_2nd -> Gear_1st [order 2] : DOWN
        Gear_5th -> Gear_4th [order 2] : DOWN
        Gear_6th -> Gear_5th [order 2] : DOWN
        Gear_7th -> Gear_6th [order 2] : DOWN
        Gear_8th -> Gear_7th : DOWN
      state Gear_Transient_D [parallel]
        du:[up_thrsh]=calc_up(Gear_D, drvAPP);
        du:[down_thrsh]=calc_down(Gear_D, drvAPP);
        settings: executionOrder=2
        state steady_state
        state upshifting
        state downshifting
        (default) -> steady_state
        steady_state -> upshifting [order 1] : [VehicleSpeed > up_thrsh && Gear_D < 8]
        steady_state -> downshifting [order 2] : [VehicleSpeed < down_thrsh && Gear_D > 1]
        downshifting -> steady_state [order 2] : [VehicleSpeed > down_thrsh]
        downshifting -> steady_state [order 1] : after(0.1,sec)
            | [VehicleSpeed <= down_thrsh]
            | {Gear_State_D.DOWN;}
        upshifting -> steady_state [order 1] : after(0.1,sec)
            | [VehicleSpeed >= up_thrsh]
            | {Gear_State_D.UP;}
        upshifting -> steady_state [order 2] : [VehicleSpeed < up_thrsh]
      state PlotShiftSchedule [function]
      state up_th = calc_up(Gear, APP) [function]
      state down_th = calc_down(Gear, APP) [function]
  data: Gear function_input; APP function_input; lockup_th function_output; Gear function_input; APP function_input; unlock_th function_output; Gear function_input; APP function_input; up_th function_output; Gear function_input; APP function_input; down_th function_output; tc_lockup_thrsh input double; Gear_D local int8 =1; drvAPP input double [0..100]; VehicleSpeed input double; TransEstGear output int8; down_thrsh local double =0; up_thrsh local double =0; LockupCmd output boolean; tc_spd_in input double; tc_spd_out input double; drvBPP input double; ShftLvrPos input int8; lockup_thrsh local double; unlock_thrsh local double
  events: DOWN local EITHER_EDGE_EVENT; UP local EITHER_EDGE_EVENT
